simulink library "GFo_Lib_R2017b"  (R2017b)
settings: Solver=VariableStepAuto  StartTime=0.0  StopTime=10.0  RelTol=1e-3
values from neighbouring files (symbols this model uses):
  Time_Step = 50e-6    (= 5e-05)    [init.m]
undefined symbols (not defined in the file or in its folder): C_line, VSC01_Cf, VSC01_id0, VSC01_Lf, VSC01_Rf
libraries: powerlib x25, Control_Lib x12, simulink x7, powerlib_meascontrol x2
(part 2 of 2)

== system GFo_Lib_R2017b/Mean Model 2-Level LCL-filter/Control loops/ pu P//Q computation ==
  v_abc_pu : Inport  PortDimensions=3
  i_abc_pu : Inport  Port=2  PortDimensions=3
  Demux : Demux  Outputs=3
      settings: DisplayOption=none
  Mux : Mux  Inputs=3
  Product1 : Product  InputSameDT=on  SaturateOnIntegerOverflow=on  OutDataTypeStr=Inherit: Same as first input
  Product3 : Product  InputSameDT=on  SaturateOnIntegerOverflow=on  OutDataTypeStr=Inherit: Same as first input
  Sum : Sum  Inputs=+-  InputSameDT=on  SaturateOnIntegerOverflow=on  OutDataTypeStr=Inherit: Same as first input
  Sum1 : Sum  Inputs=1  InputSameDT=on  SaturateOnIntegerOverflow=on  OutDataTypeStr=Inherit: Same as first input
  Sum4 : Sum  Inputs=1  InputSameDT=on  SaturateOnIntegerOverflow=on  OutDataTypeStr=Inherit: Same as first input
  Sum5 : Sum  Inputs=+-  InputSameDT=on  SaturateOnIntegerOverflow=on  OutDataTypeStr=Inherit: Same as first input
  Sum6 : Sum  Inputs=+-  InputSameDT=on  SaturateOnIntegerOverflow=on  OutDataTypeStr=Inherit: Same as first input
  pu->V : Gain  Gain=1/sqrt(3)  SaturateOnIntegerOverflow=on  OutDataTypeStr=Inherit: Same as input  ParamDataTypeStr=Inherit: Same as input
  pu->V1 : Gain  Gain=1/3  SaturateOnIntegerOverflow=on  OutDataTypeStr=Inherit: Same as input  ParamDataTypeStr=Inherit: Same as input
  pu->V2 : Gain  Gain=1/3  SaturateOnIntegerOverflow=on  OutDataTypeStr=Inherit: Same as input  ParamDataTypeStr=Inherit: Same as input
  P : Outport  VectorParamsAs1DForOutWhenUnconnected=off
  Q : Outport  Port=2  VectorParamsAs1DForOutWhenUnconnected=off
  wires:
  pu->V/1 -> pu->V2/1  "Q"
  Mux/1 -> Product3/1
  Sum6/1 -> Mux/2
  Sum5/1 -> Mux/1
  Sum/1 -> Mux/3
  Demux/3 -> Sum6/1, Sum5/2
  Demux/2 -> Sum5/1, Sum/2
  Demux/1 -> Sum6/2, Sum/1
  Sum4/1 -> pu->V1/1
  i_abc_pu/1 -> Product3/2, Product1/2
  v_abc_pu/1 -> Demux/1, Product1/1
  Product1/1 -> Sum4/1
  Product3/1 -> Sum1/1
  Sum1/1 -> pu->V/1
  pu->V1/1 -> P/1
  pu->V2/1 -> Q/1

== system GFo_Lib_R2017b/Mean Model 2-Level LCL-filter/Control loops/Damping ==
  ig_dq : Inport
  Filter w_LF : Subsystem
      mask Display: disp('\omega_{LF} / (s + \omega_{LF})','texmode','on')
  Sum5 : Sum  Inputs=|+-
  nq1 : Gain  Gain=Rv
  "Delta_E_dq " : Outport  VectorParamsAs1DForOutWhenUnconnected=off
  wires:
  ig_dq/1 -> nq1/1
  Sum5/1 -> "Delta_E_dq "/1
  Filter w_LF/1(s) -> Sum5/1
  nq1/1 -> Sum5/2, Filter w_LF/1(e)

== system GFo_Lib_R2017b/Mean Model 2-Level LCL-filter/Control loops/Inner Cascaded control loops ==
  eg_dq0_set : Inport
  eg_dq : Inport  Port=2
  ig_dq : Inport  Port=3
  is_dq : Inport  Port=4
  Amplitude : Subsystem
  Compare To Constant : simulink/Logic and Bit Operations/Compare To Constant  relop=<=  const=I_max  OutDataTypeStr=boolean
  Current PI control : Subsystem
  Memory : Memory  InitialCondition=1
  Voltage PI control : Subsystem
  w_pu : Constant
  vm_dq : Outport  VectorParamsAs1DForOutWhenUnconnected=off
  wires:
  Amplitude/2(cond) -> Compare To Constant/1
  eg_dq0_set/1 -> Voltage PI control/2(Eg_dq0_ref)
  Voltage PI control/1(Is_dq0_ref) -> Amplitude/1(is_unsat)
  Amplitude/1(is_sat) -> Current PI control/3(Is_dq0_ref)
  w_pu/1 -> Current PI control/4(w), Voltage PI control/4(w)
  Current PI control/1(Vm_dq0_ref) -> vm_dq/1
  is_dq/1 -> Current PI control/1(Is_dq0)
  eg_dq/1 -> Current PI control/2(Eg_dq0), Voltage PI control/1(Eg_dq0)
  ig_dq/1 -> Voltage PI control/3(Ig_dq0)
  Compare To Constant/1 -> Memory/1
  Memory/1 -> Voltage PI control/5(block integ)

== system GFo_Lib_R2017b/Mean Model 2-Level LCL-filter/Control loops/Power Control Loops ==
  P_mes : Inport
  P_set : Inport  Port=2
  delta_PLL : Inport  Port=3
  w_PLL : Inport  Port=4
  Compare To Constant : simulink/Logic and Bit Operations/Compare To Constant  relop===  const=1  OutDataTypeStr=boolean
  Compare To Constant1 : simulink/Logic and Bit Operations/Compare To Constant  relop===  const=2  OutDataTypeStr=boolean
  Compare To Constant2 : simulink/Logic and Bit Operations/Compare To Constant  relop===  const=3  OutDataTypeStr=boolean
  Multiport Switch : MultiPortSwitch
  Multiport Switch1 : MultiPortSwitch
  Strategy 1 : Subsystem
  Strategy 2 : Subsystem
  Strategy 3 : Subsystem
  w_set1 : Constant  Value=Chosen_Strategy
  w_set3 : Constant  Value=Chosen_Strategy
  w_set4 : Constant  Value=gainpopup
  w_set5 : Constant  Value=gainpopup
  w_set_pu : Constant
  f : Outport  VectorParamsAs1DForOutWhenUnconnected=off
  Theta : Outport  Port=2  VectorParamsAs1DForOutWhenUnconnected=off
  wires:
  P_mes/1 -> Strategy 3/1(P_mes), Strategy 2/1(P_mes), Strategy 1/1(P_mes)
  P_set/1 -> Strategy 2/2(P_set), Strategy 3/2(P_set), Strategy 1/2(P_set)
  delta_PLL/1 -> Strategy 1/3(delta_PLL)
  w_PLL/1 -> Strategy 2/3(w_PLL), Strategy 1/4(w_PLL)
  w_set_pu/1 -> Strategy 3/3(w_set_pu)
  Strategy 3/2(theta) -> Multiport Switch1/4
  Strategy 3/1(frequency) -> Multiport Switch/4
  Strategy 2/1(frequency) -> Multiport Switch/3
  w_set1/1 -> Multiport Switch1/1, Multiport Switch/1
  Strategy 2/2(theta) -> Multiport Switch1/3
  Multiport Switch1/1 -> Theta/1
  Strategy 1/2(theta) -> Multiport Switch1/2
  Multiport Switch/1 -> f/1
  Strategy 1/1(frequency) -> Multiport Switch/2
  w_set3/1 -> Compare To Constant/1
  w_set4/1 -> Compare To Constant1/1
  w_set5/1 -> Compare To Constant2/1
  Compare To Constant/1 -> Strategy 1/Enable
  Compare To Constant1/1 -> Strategy 2/Enable
  Compare To Constant2/1 -> Strategy 3/Enable

== system GFo_Lib_R2017b/Mean Model 2-Level LCL-filter/Control loops/VI ==
  note: VI
  note: VI triggering and threshold computation
  i_VI_dq : Inport
  Bus Creator : BusCreator  Inputs=1
  Demux1 : Demux  Outputs=2
      settings: DisplayOption=none
  Gain5 : Gain  Gain=DX_DR
  Gain6 : Gain  Gain=Kp_Rvi_pu
  Gain9 : Gain  Gain=DX_DR
  I_thresh : Constant  Value=I_thresh_pu
  Mux2 : Mux  Inputs=2
  Saturation : Saturate  UpperLimit=inf  LowerLimit=0
  Sum1 : Sum  Inputs=-+|
  Sum7 : Sum  Inputs=|+-
  Sum8 : Sum  Inputs=++|
  dq to phasor : Subsystem
  product{,1..3} (4 alike) : Product  InputSameDT=on  RndMeth=Zero  SaturateOnIntegerOverflow=on  OutDataTypeStr=Inherit: Same as first input
  I_rms : Outport  VectorParamsAs1DForOutWhenUnconnected=off
  Delta_E_dq : Outport  Port=2  VectorParamsAs1DForOutWhenUnconnected=off
  wires:
  i_VI_dq/1 -> Demux1/1, dq to phasor/1(dq_mes)
  Sum8/1 -> Mux2/2
  Sum7/1 -> Mux2/1
  product2/1 -> Sum8/2
  Gain9/1 -> Sum8/1
  Gain5/1 -> Sum7/2
  product1/1 -> Sum7/1
  Demux1/2 -> product3/1, product2/1  "igq"
  Demux1/1 -> product/2, product1/1  "igd"
  product/1 -> Gain9/1
  product3/1 -> Gain5/1
  Gain6/1 -> product2/2, product1/2, product/1, product3/2
  Mux2/1 -> Delta_E_dq/1
  I_thresh/1 -> Sum1/1
  Saturation/1 -> Gain6/1
  dq to phasor/1(rms) -> Bus Creator/1, Sum1/2  "I_rms"
  Sum1/1 -> Saturation/1
  Bus Creator/1 -> I_rms/1

== system GFo_Lib_R2017b/Mean Model 2-Level L-filter/Control loops/Damping/Filter w_LF ==
  e : Inport
  1/T_LP : Gain  Gain=W_TVR  SaturateOnIntegerOverflow=on  OutDataTypeStr=Inherit: Same as input  ParamDataTypeStr=Inherit: Same as input
  Integrator : Integrator  InitialConditionSource=external  InitialCondition=[VSC01_id0*0.04]
  Sum1 : Sum  Inputs=|+-  InputSameDT=on  SaturateOnIntegerOverflow=on  OutDataTypeStr=Inherit: Same as first input
  s : Outport  VectorParamsAs1DForOutWhenUnconnected=off
  wires:
  Sum1/1 -> 1/T_LP/1
  1/T_LP/1 -> Integrator/1
  Integrator/1 -> Sum1/2, s/1
  e/1 -> Integrator/2, Sum1/1

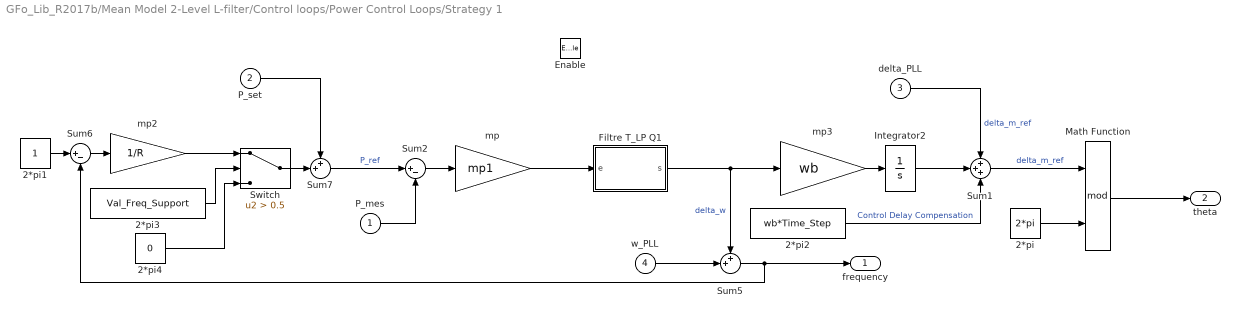
== system GFo_Lib_R2017b/Mean Model 2-Level L-filter/Control loops/Power Control Loops/Strategy 1 ==
  P_mes : Inport
  P_set : Inport  Port=2
  delta_PLL : Inport  Port=3
  w_PLL : Inport  Port=4
  Enable : EnablePort
  2*pi : Constant  Value=2*pi
  2*pi1 : Constant
  2*pi2 : Constant  Value=wb*Time_Step
  2*pi3 : Constant  Value=Val_Freq_Support
  2*pi4 : Constant  Value=0
  Filtre T_LP Q1 : Subsystem
  Integrator2 : Integrator  InitialCondition=(Theta_vsc0-Theta0)*pi/180
  Math Function : Math  Operator=mod  SaturateOnIntegerOverflow=on
  Sum1 : Sum  Inputs=+++
  Sum2 : Sum  Inputs=|+-
  Sum5 : Sum  Inputs=++|
  Sum6 : Sum  Inputs=|+-
  Sum7 : Sum  Inputs=++|
  Switch : Switch  Criteria=u2 > Threshold  Threshold=0.5
  mp : Gain  Gain=mp1
  mp2 : Gain  Gain=1/R
  mp3 : Gain  Gain=wb
  frequency : Outport  VectorParamsAs1DForOutWhenUnconnected=off
  theta : Outport  Port=2  VectorParamsAs1DForOutWhenUnconnected=off
  wires:
  Sum2/1 -> mp/1
  Sum1/1 -> Math Function/1  "delta_m_ref"
  2*pi/1 -> Math Function/2
  2*pi1/1 -> Sum6/1
  Sum6/1 -> mp2/1
  P_set/1 -> Sum7/1
  Sum7/1 -> Sum2/1  "P_ref"
  P_mes/1 -> Sum2/2
  Switch/1 -> Sum7/2
  Math Function/1 -> theta/1
  Filtre T_LP Q1/1(s) -> mp3/1, Sum5/1  "delta_w"
  mp3/1 -> Integrator2/1
  mp/1 -> Filtre T_LP Q1/1(e)
  delta_PLL/1 -> Sum1/1  "delta_m_ref"
  w_PLL/1 -> Sum5/2
  Sum5/1 -> frequency/1, Sum6/2
  2*pi2/1 -> Sum1/3  "Control Delay Compensation"
  Integrator2/1 -> Sum1/2
  mp2/1 -> Switch/1
  2*pi3/1 -> Switch/2
  2*pi4/1 -> Switch/3

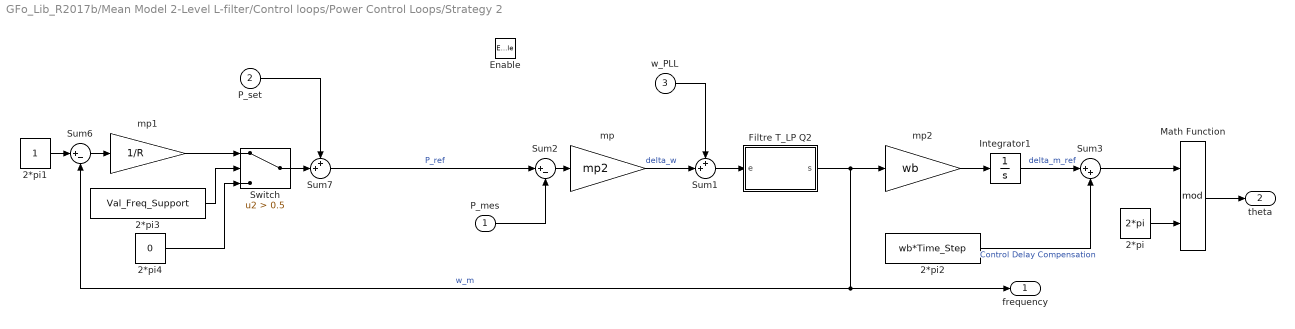
== system GFo_Lib_R2017b/Mean Model 2-Level L-filter/Control loops/Power Control Loops/Strategy 2 ==
  P_mes : Inport
  P_set : Inport  Port=2
  w_PLL : Inport  Port=3
  Enable : EnablePort
  2*pi : Constant  Value=2*pi
  2*pi1 : Constant
  2*pi2 : Constant  Value=wb*Time_Step
  2*pi3 : Constant  Value=Val_Freq_Support
  2*pi4 : Constant  Value=0
  Filtre T_LP Q2 : Subsystem
  Integrator1 : Integrator  InitialCondition=Theta_vsc0*pi/180
  Math Function : Math  Operator=mod  SaturateOnIntegerOverflow=on
  Sum1 : Sum  Inputs=++|
  Sum2 : Sum  Inputs=|+-
  Sum3 : Sum  Inputs=|++
  Sum6 : Sum  Inputs=|+-
  Sum7 : Sum  Inputs=++|
  Switch : Switch  Criteria=u2 > Threshold  Threshold=0.5
  mp : Gain  Gain=mp2
  mp1 : Gain  Gain=1/R
  mp2 : Gain  Gain=wb
  frequency : Outport  VectorParamsAs1DForOutWhenUnconnected=off
  theta : Outport  Port=2  VectorParamsAs1DForOutWhenUnconnected=off
  wires:
  Sum1/1 -> Filtre T_LP Q2/1(e)
  2*pi/1 -> Math Function/2
  Math Function/1 -> theta/1
  Integrator1/1 -> Sum3/1  "delta_m_ref"
  Sum2/1 -> mp/1
  mp/1 -> Sum1/2  "delta_w"
  Filtre T_LP Q2/1(s) -> mp2/1, frequency/1, Sum6/2  "w_m"
  w_PLL/1 -> Sum1/1
  P_mes/1 -> Sum2/2
  mp2/1 -> Integrator1/1
  2*pi2/1 -> Sum3/2  "Control Delay Compensation"
  Sum3/1 -> Math Function/1
  Switch/1 -> Sum7/2
  P_set/1 -> Sum7/1
  Sum6/1 -> mp1/1
  2*pi1/1 -> Sum6/1
  mp1/1 -> Switch/1
  2*pi3/1 -> Switch/2
  2*pi4/1 -> Switch/3
  Sum7/1 -> Sum2/1  "P_ref"

== system GFo_Lib_R2017b/Mean Model 2-Level L-filter/Control loops/Power Control Loops/Strategy 3 ==
  P_mes : Inport
  P_set : Inport  Port=2
  w_set_pu : Inport  Port=3
  Enable : EnablePort
  2*pi : Constant  Value=2*pi
  2*pi2 : Constant  Value=wb*Time_Step
  Filtre T_LP Q2 : Subsystem
  Integrator1 : Integrator  InitialCondition=Theta_vsc0*pi/180
  Lead-Lag Filter : powerlib_meascontrol/Filters/Lead-Lag Filter  T1=T1  T2=T2  Vdc_Init=P0  Ts=0
      settings: SourceProductBaseCode=PS
  Math Function : Math  Operator=mod  SaturateOnIntegerOverflow=on
  Sum1 : Sum  Inputs=++|
  Sum2 : Sum  Inputs=|+-
  Sum3 : Sum  Inputs=|++
  mp : Gain  Gain=mp3
  mp1 : Gain  Gain=wb
  frequency : Outport  VectorParamsAs1DForOutWhenUnconnected=off
  theta : Outport  Port=2  VectorParamsAs1DForOutWhenUnconnected=off
  wires:
  Sum2/1 -> mp/1
  Integrator1/1 -> Sum3/1  "delta_m_ref"
  Math Function/1 -> theta/1
  2*pi/1 -> Math Function/2
  w_set_pu/1 -> Sum1/1
  P_set/1 -> Sum2/1
  mp/1 -> Sum1/2  "delta_w"
  Filtre T_LP Q2/1(s) -> frequency/1, mp1/1
  P_mes/1 -> Lead-Lag Filter/1
  Sum1/1 -> Filtre T_LP Q2/1(e)
  mp1/1 -> Integrator1/1  "w_m"
  Sum3/1 -> Math Function/1
  2*pi2/1 -> Sum3/2  "Control Delay Compensation"
  Lead-Lag Filter/1 -> Sum2/2

== system GFo_Lib_R2017b/Mean Model 2-Level L-filter/Control loops/VI/dq to phasor ==
  dq_mes : Inport
  Demux : Demux  Outputs=2
      settings: DisplayOption=none
  Sqrt : Sqrt  SaturateOnIntegerOverflow=on
  Sum4 : Sum  Inputs=|++  InputSameDT=on  SaturateOnIntegerOverflow=on  OutDataTypeStr=Inherit: Same as first input
  Vrdird : Product  InputSameDT=on  RndMeth=Zero  SaturateOnIntegerOverflow=on  OutDataTypeStr=Inherit: Same as first input
  Vrqirq : Product  InputSameDT=on  RndMeth=Zero  SaturateOnIntegerOverflow=on  OutDataTypeStr=Inherit: Same as first input
  rms : Outport  VectorParamsAs1DForOutWhenUnconnected=off
  wires:
  Sqrt/1 -> rms/1
  dq_mes/1 -> Demux/1
  Demux/1 -> Vrdird/1, Vrdird/2
  Demux/2 -> Vrqirq/1, Vrqirq/2
  Vrdird/1 -> Sum4/1
  Vrqirq/1 -> Sum4/2
  Sum4/1 -> Sqrt/1

== system GFo_Lib_R2017b/Mean Model 2-Level LCL-filter/Control loops/Damping/Filter w_LF ==
  e : Inport
  1/T_LP : Gain  Gain=W_TVR  SaturateOnIntegerOverflow=on  OutDataTypeStr=Inherit: Same as input  ParamDataTypeStr=Inherit: Same as input
  Integrator : Integrator  InitialConditionSource=external  InitialCondition=[VSC01_id0*0.04]
  Sum1 : Sum  Inputs=|+-  InputSameDT=on  SaturateOnIntegerOverflow=on  OutDataTypeStr=Inherit: Same as first input
  s : Outport  VectorParamsAs1DForOutWhenUnconnected=off
  wires:
  Sum1/1 -> 1/T_LP/1
  1/T_LP/1 -> Integrator/1
  Integrator/1 -> Sum1/2, s/1
  e/1 -> Integrator/2, Sum1/1

== system GFo_Lib_R2017b/Mean Model 2-Level LCL-filter/Control loops/Inner Cascaded control loops/Amplitude ==
  is_unsat : Inport
  Saturation2 : Saturate  UpperLimit=I_max  LowerLimit=0
  Source Element3 : Subsystem
  Subsystem : Subsystem
  dq to phasor : Subsystem
  is_sat : Outport  VectorParamsAs1DForOutWhenUnconnected=off
  cond : Outport  Port=2  VectorParamsAs1DForOutWhenUnconnected=off
  wires:
  dq to phasor/1(rms) -> cond/1, Saturation2/1
  Source Element3/1(ig_sat) -> is_sat/1
  Saturation2/1 -> Source Element3/1(Is_sat)
  Subsystem/1(phi) -> Source Element3/2(phi)
  is_unsat/1 -> dq to phasor/1(dq_mes), Subsystem/1(is_unsat)

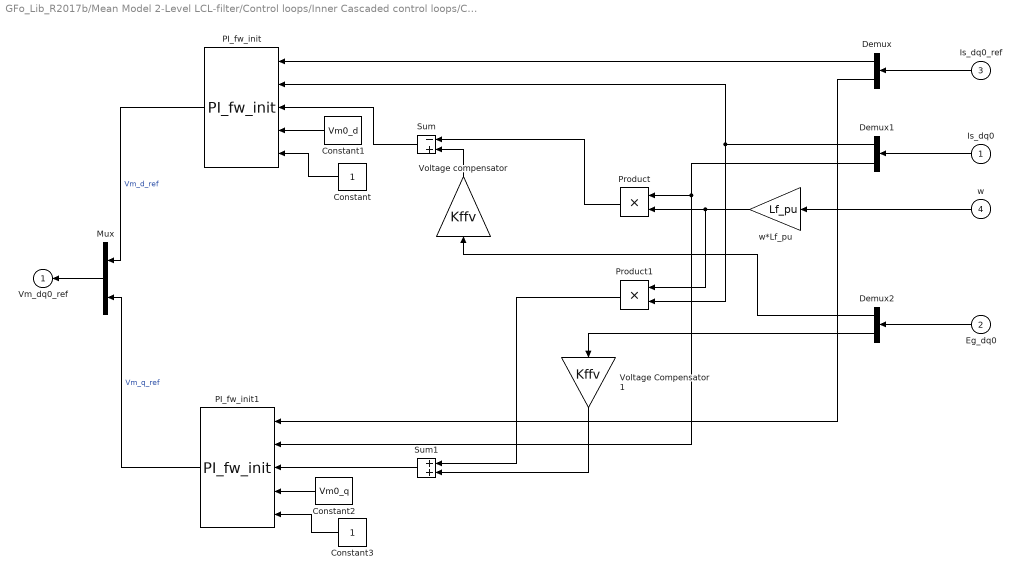
== system GFo_Lib_R2017b/Mean Model 2-Level LCL-filter/Control loops/Inner Cascaded control loops/Current PI control ==
  Is_dq0 : Inport
  Eg_dq0 : Inport  Port=2
  Is_dq0_ref : Inport  Port=3
  w : Inport  Port=4
  Constant : Constant
  Constant1 : Constant  Value=Vm0_d
  Constant2 : Constant  Value=Vm0_q
  Constant3 : Constant
  Demux : Demux  Outputs=2
  Demux1 : Demux  Outputs=2
  Demux2 : Demux  Outputs=2
  Mux : Mux  Inputs=[1 1]
  PI_fw_init : Control_Lib/PI_fw_init  Kp=Kp_i  Ki=Ki_i
      settings: SourceProductName=VSC4SPS
  PI_fw_init1 : Control_Lib/PI_fw_init  Kp=Kp_i  Ki=Ki_i
      settings: SourceProductName=VSC4SPS
  Product : Product  RndMeth=Zero
  Product1 : Product  RndMeth=Zero
  Sum : Sum  Inputs=-+
  Sum1 : Sum
  Voltage Compensator 1 : Gain  Gain=Kffv
  Voltage compensator : Gain  Gain=Kffv
  w*Lf_pu : Gain  Gain=Lf_pu
  Vm_dq0_ref : Outport  InitialOutput=0  VectorParamsAs1DForOutWhenUnconnected=off
  wires:
  Voltage compensator/1 -> Sum/2
  w/1 -> w*Lf_pu/1
  PI_fw_init1/1 -> Mux/2  "Vm_q_ref"
  PI_fw_init/1 -> Mux/1  "Vm_d_ref"
  Product1/1 -> Sum1/1
  Demux/2 -> PI_fw_init1/1
  Mux/1 -> Vm_dq0_ref/1
  Demux1/2 -> PI_fw_init1/2, Product/1
  w*Lf_pu/1 -> Product/2, Product1/1
  Demux1/1 -> PI_fw_init/2, Product1/2
  Demux/1 -> PI_fw_init/1
  Is_dq0_ref/1 -> Demux/1
  Is_dq0/1 -> Demux1/1
  Demux2/1 -> Voltage compensator/1
  Demux2/2 -> Voltage Compensator 1/1
  Eg_dq0/1 -> Demux2/1
  Product/1 -> Sum/1
  Sum/1 -> PI_fw_init/3
  Constant/1 -> PI_fw_init/5
  Constant1/1 -> PI_fw_init/4
  Sum1/1 -> PI_fw_init1/3
  Voltage Compensator 1/1 -> Sum1/2
  Constant2/1 -> PI_fw_init1/4
  Constant3/1 -> PI_fw_init1/5

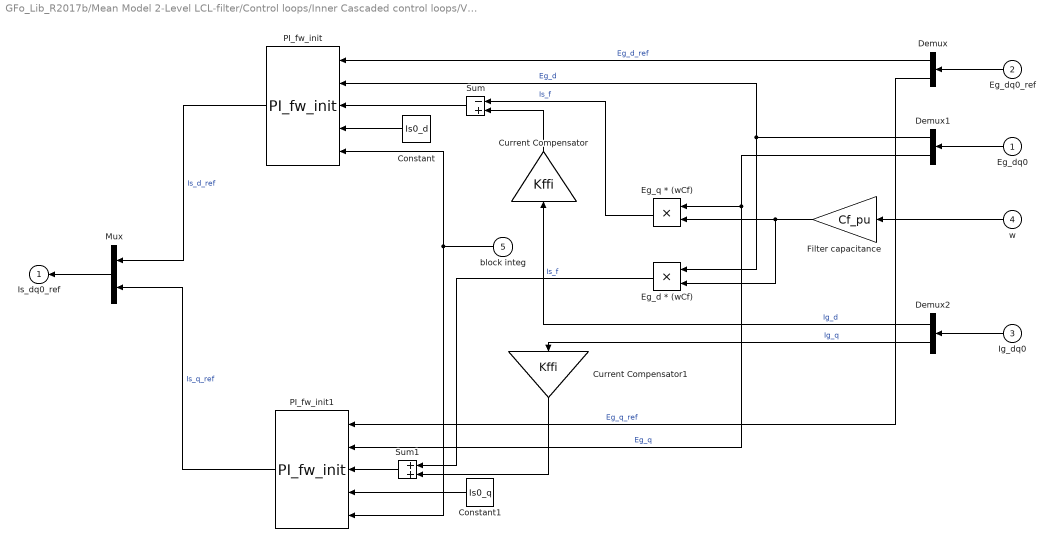
== system GFo_Lib_R2017b/Mean Model 2-Level LCL-filter/Control loops/Inner Cascaded control loops/Voltage PI control ==
  Eg_dq0 : Inport
  Eg_dq0_ref : Inport  Port=2
  Ig_dq0 : Inport  Port=3
  w : Inport  Port=4
  block integ : Inport  Port=5
  Constant : Constant  Value=Is0_d
  Constant1 : Constant  Value=Is0_q
  Current Compensator : Gain  Gain=Kffi
  Current Compensator1 : Gain  Gain=Kffi
  Demux : Demux  Outputs=2
  Demux1 : Demux  Outputs=2
  Demux2 : Demux  Outputs=2
  Eg_d * (wCf) : Product  RndMeth=Zero
  "Eg_q * (wCf) " : Product  RndMeth=Zero
  Filter capacitance : Gain  Gain=Cf_pu
  Mux : Mux  Inputs=2
  PI_fw_init : Control_Lib/PI_fw_init  Kp=Kp_v  Ki=Ki_v
      settings: SourceProductName=VSC4SPS
  PI_fw_init1 : Control_Lib/PI_fw_init  Kp=Kp_v  Ki=Ki_v
      settings: SourceProductName=VSC4SPS
  Sum : Sum  Inputs=-+
  Sum1 : Sum
  Is_dq0_ref : Outport  InitialOutput=0  VectorParamsAs1DForOutWhenUnconnected=off
  wires:
  block integ/1 -> PI_fw_init1/5, PI_fw_init/5
  Current Compensator1/1 -> Sum1/2
  w/1 -> Filter capacitance/1
  PI_fw_init/1 -> Mux/1  "Is_d_ref"
  Demux2/2 -> Current Compensator1/1  "Ig_q"
  Eg_d * (wCf)/1 -> Sum1/1  "Is_f"
  Demux/2 -> PI_fw_init1/1  "Eg_q_ref"
  Mux/1 -> Is_dq0_ref/1
  Demux2/1 -> Current Compensator/1  "Ig_d"
  "Eg_q * (wCf) "/1 -> Sum/1  "Is_f"
  Demux1/2 -> PI_fw_init1/2, "Eg_q * (wCf) "/1  "Eg_q"
  Filter capacitance/1 -> Eg_d * (wCf)/2, "Eg_q * (wCf) "/2
  Demux1/1 -> PI_fw_init/2, Eg_d * (wCf)/1  "Eg_d"
  Demux/1 -> PI_fw_init/1  "Eg_d_ref"
  Eg_dq0/1 -> Demux1/1
  Eg_dq0_ref/1 -> Demux/1
  Ig_dq0/1 -> Demux2/1
  Sum/1 -> PI_fw_init/3
  Current Compensator/1 -> Sum/2
  Constant/1 -> PI_fw_init/4
  Sum1/1 -> PI_fw_init1/3
  PI_fw_init1/1 -> Mux/2  "Is_q_ref"
  Constant1/1 -> PI_fw_init1/4

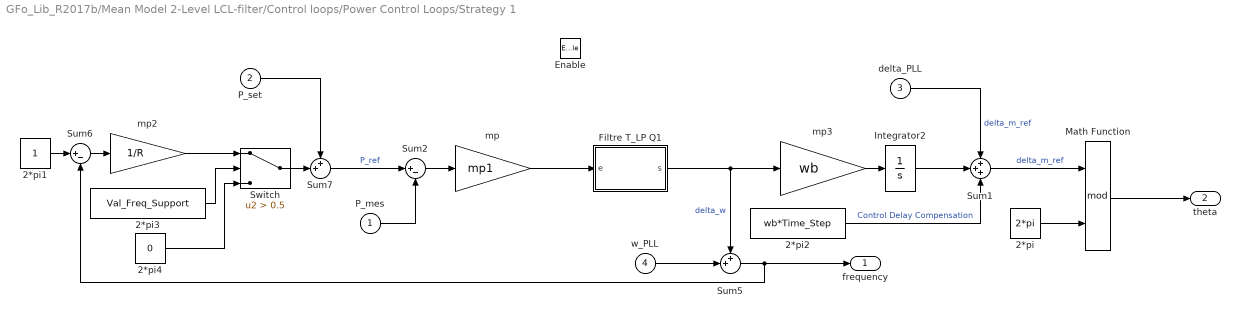
== system GFo_Lib_R2017b/Mean Model 2-Level LCL-filter/Control loops/Power Control Loops/Strategy 1 ==
  P_mes : Inport
  P_set : Inport  Port=2
  delta_PLL : Inport  Port=3
  w_PLL : Inport  Port=4
  Enable : EnablePort
  2*pi : Constant  Value=2*pi
  2*pi1 : Constant
  2*pi2 : Constant  Value=wb*Time_Step
  2*pi3 : Constant  Value=Val_Freq_Support
  2*pi4 : Constant  Value=0
  Filtre T_LP Q1 : Subsystem
  Integrator2 : Integrator  InitialCondition=(Theta_m0)*pi/180-Theta0*pi/180
  Math Function : Math  Operator=mod  SaturateOnIntegerOverflow=on
  Sum1 : Sum  Inputs=+++
  Sum2 : Sum  Inputs=|+-
  Sum5 : Sum  Inputs=++|
  Sum6 : Sum  Inputs=|+-
  Sum7 : Sum  Inputs=++|
  Switch : Switch  Criteria=u2 > Threshold  Threshold=0.5
  mp : Gain  Gain=mp1
  mp2 : Gain  Gain=1/R
  mp3 : Gain  Gain=wb
  frequency : Outport  VectorParamsAs1DForOutWhenUnconnected=off
  theta : Outport  Port=2  VectorParamsAs1DForOutWhenUnconnected=off
  wires:
  Sum2/1 -> mp/1
  Sum1/1 -> Math Function/1  "delta_m_ref"
  2*pi/1 -> Math Function/2
  2*pi1/1 -> Sum6/1
  Sum6/1 -> mp2/1
  P_set/1 -> Sum7/1
  Sum7/1 -> Sum2/1  "P_ref"
  P_mes/1 -> Sum2/2
  Switch/1 -> Sum7/2
  Math Function/1 -> theta/1
  Filtre T_LP Q1/1(s) -> mp3/1, Sum5/1  "delta_w"
  mp3/1 -> Integrator2/1
  mp/1 -> Filtre T_LP Q1/1(e)
  delta_PLL/1 -> Sum1/1  "delta_m_ref"
  w_PLL/1 -> Sum5/2
  Sum5/1 -> frequency/1, Sum6/2
  2*pi2/1 -> Sum1/3  "Control Delay Compensation"
  Integrator2/1 -> Sum1/2
  mp2/1 -> Switch/1
  2*pi3/1 -> Switch/2
  2*pi4/1 -> Switch/3

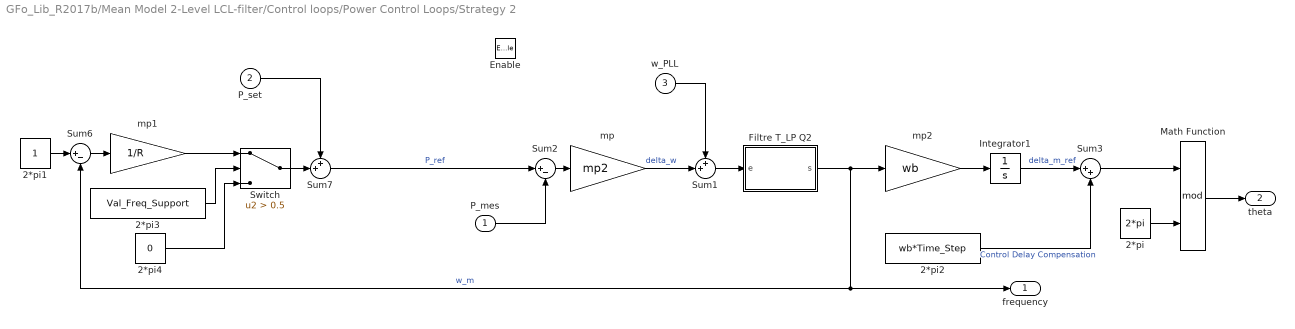
== system GFo_Lib_R2017b/Mean Model 2-Level LCL-filter/Control loops/Power Control Loops/Strategy 2 ==
  P_mes : Inport
  P_set : Inport  Port=2
  w_PLL : Inport  Port=3
  Enable : EnablePort
  2*pi : Constant  Value=2*pi
  2*pi1 : Constant
  2*pi2 : Constant  Value=wb*Time_Step
  2*pi3 : Constant  Value=Val_Freq_Support
  2*pi4 : Constant  Value=0
  Filtre T_LP Q2 : Subsystem
  Integrator1 : Integrator  InitialCondition=Theta_m0*pi/180
  Math Function : Math  Operator=mod  SaturateOnIntegerOverflow=on
  Sum1 : Sum  Inputs=++|
  Sum2 : Sum  Inputs=|+-
  Sum3 : Sum  Inputs=|++
  Sum6 : Sum  Inputs=|+-
  Sum7 : Sum  Inputs=++|
  Switch : Switch  Criteria=u2 > Threshold  Threshold=0.5
  mp : Gain  Gain=mp2
  mp1 : Gain  Gain=1/R
  mp2 : Gain  Gain=wb
  frequency : Outport  VectorParamsAs1DForOutWhenUnconnected=off
  theta : Outport  Port=2  VectorParamsAs1DForOutWhenUnconnected=off
  wires:
  Sum1/1 -> Filtre T_LP Q2/1(e)
  2*pi/1 -> Math Function/2
  Math Function/1 -> theta/1
  Integrator1/1 -> Sum3/1  "delta_m_ref"
  Sum2/1 -> mp/1
  mp/1 -> Sum1/2  "delta_w"
  Filtre T_LP Q2/1(s) -> mp2/1, frequency/1, Sum6/2  "w_m"
  w_PLL/1 -> Sum1/1
  P_mes/1 -> Sum2/2
  mp2/1 -> Integrator1/1
  2*pi2/1 -> Sum3/2  "Control Delay Compensation"
  Sum3/1 -> Math Function/1
  Switch/1 -> Sum7/2
  P_set/1 -> Sum7/1
  Sum6/1 -> mp1/1
  2*pi1/1 -> Sum6/1
  mp1/1 -> Switch/1
  2*pi3/1 -> Switch/2
  2*pi4/1 -> Switch/3
  Sum7/1 -> Sum2/1  "P_ref"

== system GFo_Lib_R2017b/Mean Model 2-Level LCL-filter/Control loops/Power Control Loops/Strategy 3 ==
  P_mes : Inport
  P_set : Inport  Port=2
  w_set_pu : Inport  Port=3
  Enable : EnablePort
  2*pi : Constant  Value=2*pi
  2*pi2 : Constant  Value=wb*Time_Step
  Filtre T_LP Q2 : Subsystem
  Integrator1 : Integrator  InitialCondition=(Theta_m0)*pi/180
  Lead-Lag Filter : powerlib_meascontrol/Filters/Lead-Lag Filter  T1=T1  T2=T2  Vdc_Init=P0  Ts=0
      settings: SourceProductBaseCode=PS
  Math Function : Math  Operator=mod  SaturateOnIntegerOverflow=on
  Sum1 : Sum  Inputs=++|
  Sum2 : Sum  Inputs=|+-
  Sum3 : Sum  Inputs=|++
  mp : Gain  Gain=mp3
  mp1 : Gain  Gain=wb
  frequency : Outport  VectorParamsAs1DForOutWhenUnconnected=off
  theta : Outport  Port=2  VectorParamsAs1DForOutWhenUnconnected=off
  wires:
  Sum2/1 -> mp/1
  Integrator1/1 -> Sum3/1  "delta_m_ref"
  Math Function/1 -> theta/1
  2*pi/1 -> Math Function/2
  w_set_pu/1 -> Sum1/1
  P_set/1 -> Sum2/1
  mp/1 -> Sum1/2  "delta_w"
  Filtre T_LP Q2/1(s) -> frequency/1, mp1/1
  P_mes/1 -> Lead-Lag Filter/1
  Sum1/1 -> Filtre T_LP Q2/1(e)
  mp1/1 -> Integrator1/1  "w_m"
  Sum3/1 -> Math Function/1
  2*pi2/1 -> Sum3/2  "Control Delay Compensation"
  Lead-Lag Filter/1 -> Sum2/2

== system GFo_Lib_R2017b/Mean Model 2-Level LCL-filter/Control loops/VI/dq to phasor ==
  dq_mes : Inport
  Demux : Demux  Outputs=2
      settings: DisplayOption=none
  Sqrt : Sqrt  SaturateOnIntegerOverflow=on
  Sum4 : Sum  Inputs=|++  InputSameDT=on  SaturateOnIntegerOverflow=on  OutDataTypeStr=Inherit: Same as first input
  Vrdird : Product  InputSameDT=on  RndMeth=Zero  SaturateOnIntegerOverflow=on  OutDataTypeStr=Inherit: Same as first input
  Vrqirq : Product  InputSameDT=on  RndMeth=Zero  SaturateOnIntegerOverflow=on  OutDataTypeStr=Inherit: Same as first input
  rms : Outport  VectorParamsAs1DForOutWhenUnconnected=off
  wires:
  Sqrt/1 -> rms/1
  dq_mes/1 -> Demux/1
  Demux/1 -> Vrdird/1, Vrdird/2
  Demux/2 -> Vrqirq/1, Vrqirq/2
  Vrdird/1 -> Sum4/1
  Vrqirq/1 -> Sum4/2
  Sum4/1 -> Sqrt/1

== system GFo_Lib_R2017b/Mean Model 2-Level L-filter/Control loops/Power Control Loops/Strategy 1/Filtre T_LP Q1 ==
  e : Inport
  1/T_LP : Gain  Gain=wc1  SaturateOnIntegerOverflow=on  OutDataTypeStr=Inherit: Same as input  ParamDataTypeStr=Inherit: Same as input
  Integrator : Integrator
  Sum1 : Sum  Inputs=|+-  InputSameDT=on  SaturateOnIntegerOverflow=on  OutDataTypeStr=Inherit: Same as first input
  s : Outport  VectorParamsAs1DForOutWhenUnconnected=off
  wires:
  Sum1/1 -> 1/T_LP/1
  1/T_LP/1 -> Integrator/1
  Integrator/1 -> Sum1/2, s/1
  e/1 -> Sum1/1

== system GFo_Lib_R2017b/Mean Model 2-Level L-filter/Control loops/Power Control Loops/Strategy 2/Filtre T_LP Q2 ==
  e : Inport
  1/T_LP : Gain  Gain=wc2  SaturateOnIntegerOverflow=on  OutDataTypeStr=Inherit: Same as input  ParamDataTypeStr=Inherit: Same as input
  Integrator : Integrator  InitialCondition=1
  Sum1 : Sum  Inputs=|+-  InputSameDT=on  SaturateOnIntegerOverflow=on  OutDataTypeStr=Inherit: Same as first input
  s : Outport  VectorParamsAs1DForOutWhenUnconnected=off
  wires:
  Sum1/1 -> 1/T_LP/1
  1/T_LP/1 -> Integrator/1
  Integrator/1 -> Sum1/2, s/1
  e/1 -> Sum1/1

== system GFo_Lib_R2017b/Mean Model 2-Level L-filter/Control loops/Power Control Loops/Strategy 3/Filtre T_LP Q2 ==
  e : Inport
  1/T_LP : Gain  Gain=wc3  SaturateOnIntegerOverflow=on  OutDataTypeStr=Inherit: Same as input  ParamDataTypeStr=Inherit: Same as input
  Integrator : Integrator  InitialCondition=1
  Sum1 : Sum  Inputs=|+-  InputSameDT=on  SaturateOnIntegerOverflow=on  OutDataTypeStr=Inherit: Same as first input
  s : Outport  VectorParamsAs1DForOutWhenUnconnected=off
  wires:
  Sum1/1 -> 1/T_LP/1
  1/T_LP/1 -> Integrator/1
  Integrator/1 -> Sum1/2, s/1
  e/1 -> Sum1/1

== system GFo_Lib_R2017b/Mean Model 2-Level LCL-filter/Control loops/Inner Cascaded control loops/Amplitude/Source Element3 ==
  Is_sat : Inport
  phi : Inport  Port=2
  Mux : Mux  Inputs=2
  Product : Product
  Product1 : Product
  Trigonometric Function : Trigonometry  Operator=cos
  Trigonometric Function1 : Trigonometry
  ig_sat : Outport  InitialOutput=0  VectorParamsAs1DForOutWhenUnconnected=off
  wires:
  Is_sat/1 -> Product1/1, Product/1
  phi/1 -> Trigonometric Function1/1, Trigonometric Function/1
  Product/1 -> Mux/1
  Product1/1 -> Mux/2
  Mux/1 -> ig_sat/1
  Trigonometric Function1/1 -> Product1/2
  Trigonometric Function/1 -> Product/2

== system GFo_Lib_R2017b/Mean Model 2-Level LCL-filter/Control loops/Inner Cascaded control loops/Amplitude/Subsystem ==
  is_unsat : Inport
  Demux2 : Demux  Outputs=2
  Trigonometric Function : Trigonometry  Operator=atan2  NumberOfIterations=5  OutputSignalType=real
  phi : Outport  VectorParamsAs1DForOutWhenUnconnected=off
  wires:
  Demux2/2 -> Trigonometric Function/1
  Trigonometric Function/1 -> phi/1
  Demux2/1 -> Trigonometric Function/2
  is_unsat/1 -> Demux2/1

== system GFo_Lib_R2017b/Mean Model 2-Level LCL-filter/Control loops/Inner Cascaded control loops/Amplitude/dq to phasor ==
  dq_mes : Inport
  Demux : Demux  Outputs=2
      settings: DisplayOption=none
  Sqrt : Sqrt  SaturateOnIntegerOverflow=on
  Sum4 : Sum  Inputs=|++  InputSameDT=on  SaturateOnIntegerOverflow=on  OutDataTypeStr=Inherit: Same as first input
  Vrdird : Product  InputSameDT=on  RndMeth=Zero  SaturateOnIntegerOverflow=on  OutDataTypeStr=Inherit: Same as first input
  Vrqirq : Product  InputSameDT=on  RndMeth=Zero  SaturateOnIntegerOverflow=on  OutDataTypeStr=Inherit: Same as first input
  rms : Outport  VectorParamsAs1DForOutWhenUnconnected=off
  wires:
  Sqrt/1 -> rms/1
  dq_mes/1 -> Demux/1
  Demux/1 -> Vrdird/1, Vrdird/2
  Demux/2 -> Vrqirq/1, Vrqirq/2
  Vrdird/1 -> Sum4/1
  Vrqirq/1 -> Sum4/2
  Sum4/1 -> Sqrt/1

== system GFo_Lib_R2017b/Mean Model 2-Level LCL-filter/Control loops/Power Control Loops/Strategy 1/Filtre T_LP Q1 ==
  e : Inport
  1/T_LP : Gain  Gain=wc1  SaturateOnIntegerOverflow=on  OutDataTypeStr=Inherit: Same as input  ParamDataTypeStr=Inherit: Same as input
  Integrator : Integrator
  Sum1 : Sum  Inputs=|+-  InputSameDT=on  SaturateOnIntegerOverflow=on  OutDataTypeStr=Inherit: Same as first input
  s : Outport  VectorParamsAs1DForOutWhenUnconnected=off
  wires:
  Sum1/1 -> 1/T_LP/1
  1/T_LP/1 -> Integrator/1
  Integrator/1 -> Sum1/2, s/1
  e/1 -> Sum1/1

== system GFo_Lib_R2017b/Mean Model 2-Level LCL-filter/Control loops/Power Control Loops/Strategy 2/Filtre T_LP Q2 ==
  e : Inport
  1/T_LP : Gain  Gain=wc2  SaturateOnIntegerOverflow=on  OutDataTypeStr=Inherit: Same as input  ParamDataTypeStr=Inherit: Same as input
  Integrator : Integrator  InitialCondition=1
  Sum1 : Sum  Inputs=|+-  InputSameDT=on  SaturateOnIntegerOverflow=on  OutDataTypeStr=Inherit: Same as first input
  s : Outport  VectorParamsAs1DForOutWhenUnconnected=off
  wires:
  Sum1/1 -> 1/T_LP/1
  1/T_LP/1 -> Integrator/1
  Integrator/1 -> Sum1/2, s/1
  e/1 -> Sum1/1

== system GFo_Lib_R2017b/Mean Model 2-Level LCL-filter/Control loops/Power Control Loops/Strategy 3/Filtre T_LP Q2 ==
  e : Inport
  1/T_LP : Gain  Gain=wc3  SaturateOnIntegerOverflow=on  OutDataTypeStr=Inherit: Same as input  ParamDataTypeStr=Inherit: Same as input
  Integrator : Integrator  InitialCondition=1
  Sum1 : Sum  Inputs=|+-  InputSameDT=on  SaturateOnIntegerOverflow=on  OutDataTypeStr=Inherit: Same as first input
  s : Outport  VectorParamsAs1DForOutWhenUnconnected=off
  wires:
  Sum1/1 -> 1/T_LP/1
  1/T_LP/1 -> Integrator/1
  Integrator/1 -> Sum1/2, s/1
  e/1 -> Sum1/1
